simulink model "Navigation_loop_Animation"  (Simulink 8.5)
settings: Solver=ode45  StartTime=0.0  StopTime=20  RelTol=1e-3
values from neighbouring files (symbols this model uses):
  g = 9.8    [init_pararmeters.m]
  kdp = 0.4    [init_pararmeters.m]
  kdps = 0.4    [init_pararmeters.m]
  kdt = 0.4    [init_pararmeters.m]
  kdx = 0.5    [init_pararmeters.m]
  kdy = 0.5    [init_pararmeters.m]
  kdz = 20    [init_pararmeters.m]
  kix = 0    [init_pararmeters.m]
  kiy = 0    [init_pararmeters.m]
  kpp = 0.8    [init_pararmeters.m]
  kpps = 1    [init_pararmeters.m]
  kpt = 1.2    [init_pararmeters.m]
  kpx = 0.8    [init_pararmeters.m]
  kpy = 0.8    [init_pararmeters.m]
  kpz = 100    [init_pararmeters.m]
libraries: aerolibutil x2, vrlib x1
settings Model: Creator=abdelrazzak.merheb  LastModifiedBy=flying
settings DebuggingCC: SolverPrmCheckMsg=warning  FcnCallInpInsideContextMsg=UseLocalSettings

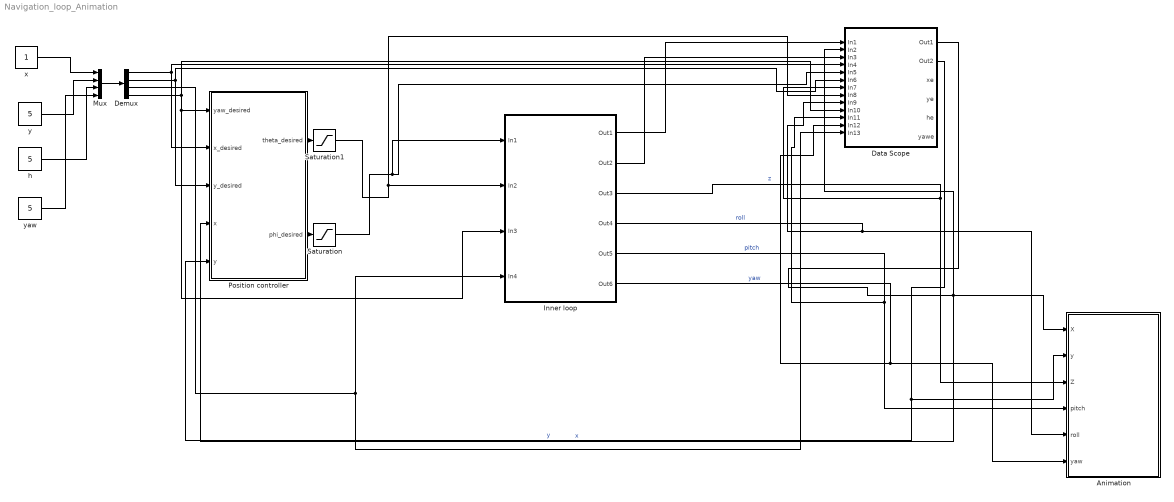
== system Navigation_loop_Animation ==
  "Animation " : Subsystem
  Data Scope : Subsystem
  Demux : Demux
  Inner loop : Subsystem
  Mux : Mux
  Position controller : Subsystem
  Saturation : Saturate  UpperLimit=35/57.3  LowerLimit=-35/57.3
  Saturation1 : Saturate  UpperLimit=35/57.3  LowerLimit=-35/57.3
  h : Constant  Value=5
  x : Constant
  y : Constant  Value=5
  yaw : Constant  Value=5
  wires:
  Demux/3 -> Inner loop/4(In4), Data Scope/13(In13)
  Demux/4 -> Data Scope/10(In10), Inner loop/3(In3), Position controller/1(yaw_desired)
  Demux/1 -> Data Scope/4(In4), Position controller/2(x_desired)
  Demux/2 -> Data Scope/6(In6), Position controller/3(y_desired)
  Saturation/1 -> Inner loop/1(In1), Data Scope/5(In5)
  Saturation1/1 -> Data Scope/8(In8), Inner loop/2(In2)
  Position controller/1(theta_desired) -> Saturation1/1
  Position controller/2(phi_desired) -> Saturation/1
  Data Scope/1(Out1) -> "Animation "/1(X), Data Scope/2(In2), Position controller/4(x)  "x"
  Data Scope/2(Out2) -> Position controller/5(y), "Animation "/2(y)  "y"
  Inner loop/5(Out5) -> "Animation "/4(pitch), Data Scope/11(In11)  "pitch"
  Inner loop/3(Out3) -> "Animation "/3(Z), Data Scope/7(In7)  "z"
  Inner loop/4(Out4) -> "Animation "/5(roll), Data Scope/9(In9)  "roll"
  Inner loop/6(Out6) -> "Animation "/6(yaw), Data Scope/12(In12)  "yaw"
  Inner loop/1(Out1) -> Data Scope/1(In1)
  Inner loop/2(Out2) -> Data Scope/3(In3)
  Mux/1 -> Demux/1
  x/1 -> Mux/1
  y/1 -> Mux/2
  h/1 -> Mux/3
  yaw/1 -> Mux/4

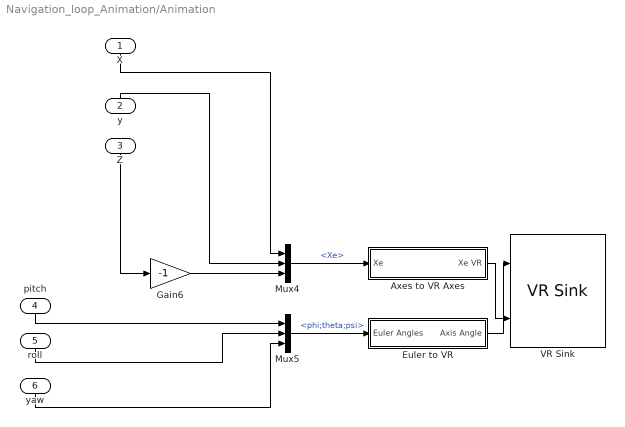
== system Navigation_loop_Animation/Animation  ==
  X : Inport
  y : Inport  Port=2
  Z : Inport  Port=3
  pitch : Inport  Port=4
  roll : Inport  Port=5
  yaw : Inport  Port=6
  Axes to VR Axes : Subsystem
  Euler to VR : Subsystem
  Gain6 : Gain  Gain=-1
  Mux4 : Mux  Inputs=3
  Mux5 : Mux  Inputs=3
  VR Sink : vrlib/VR Sink  InstantiateOnLoad=on  SampleTime=0.1  ViewEnable=on  RemoteChange=off  RemoteView=on  FieldsWritten=MyAirCraft.rotation.4.1.1.double#MyAirCraft.translation.3.1.1.double  WorldFileName=rollTst.wrl  AutoView=off  VideoDimensions=[]  AllowVariableSize=off
  wires:
  Mux5/1 -> Euler to VR/1(Euler Angles)  "<phi;theta;psi>"
  Gain6/1 -> Mux4/3
  Axes to VR Axes/1(Xe VR) -> VR Sink/2
  Euler to VR/1(Axis Angle) -> VR Sink/1
  Mux4/1 -> Axes to VR Axes/1(Xe)  "<Xe>"
  yaw/1 -> Mux5/3
  roll/1 -> Mux5/2
  y/1 -> Mux4/2
  pitch/1 -> Mux5/1
  Z/1 -> Gain6/1
  X/1 -> Mux4/1

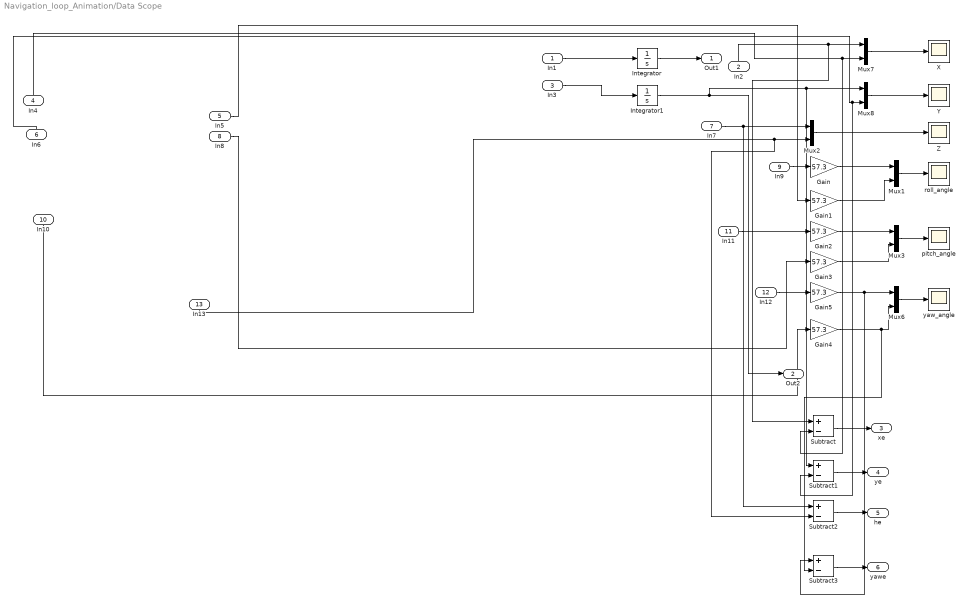
== system Navigation_loop_Animation/Data Scope ==
  In1 : Inport
  In2 : Inport  Port=2
  In3 : Inport  Port=3
  In4 : Inport  Port=4
  In5 : Inport  Port=5
  In6 : Inport  Port=6
  In7 : Inport  Port=7
  In8 : Inport  Port=8
  In9 : Inport  Port=9
  In10 : Inport  Port=10
  In11 : Inport  Port=11
  In12 : Inport  Port=12
  In13 : Inport  Port=13
  Gain{,1..5} (6 alike) : Gain  Gain=57.3
  Integrator : Integrator
  Integrator1 : Integrator
  Mux{1..3,6..8} (6 alike) : Mux  Inputs=2
  Subtract{,1..3} (4 alike) : Sum  Inputs=+-
  X : Scope
      settings: YMin=9.50171  YMax=10.5019
  Y : Scope
      settings: YMin=-53000  YMax=-50750  SaveName=ScopeData2
  Z : Scope
      settings: YMin=95  YMax=105  SaveName=ScopeData3
  pitch_angle : Scope
  roll_angle : Scope
      settings: YMax=20  SaveName=ScopeData4
  yaw_angle : Scope
      settings: YMin=-3.29867  YMax=-2.98451  SaveName=ScopeData5
  Out1 : Outport
  Out2 : Outport  Port=2
  xe : Outport  Port=3
  ye : Outport  Port=4
  he : Outport  Port=5
  yawe : Outport  Port=6
  wires:
  In1/1 -> Integrator/1
  Integrator1/1 -> Out2/1, Mux8/1, Subtract1/1
  Mux1/1 -> roll_angle/1
  In3/1 -> Integrator1/1
  Integrator/1 -> Out1/1
  Gain/1 -> Mux1/1
  Gain5/1 -> Subtract3/1, Mux6/1
  Gain4/1 -> Subtract3/2, Mux6/2
  Mux8/1 -> Y/1
  Mux7/1 -> X/1
  Gain3/1 -> Mux3/2
  Mux3/1 -> pitch_angle/1
  Mux2/1 -> Z/1
  Gain1/1 -> Mux1/2
  Gain2/1 -> Mux3/1
  Mux6/1 -> yaw_angle/1
  In12/1 -> Gain5/1
  In9/1 -> Gain/1
  In2/1 -> Subtract/1, Mux7/1
  In11/1 -> Gain2/1
  In8/1 -> Gain3/1
  In13/1 -> Subtract2/2, Mux2/2
  In5/1 -> Gain1/1
  In4/1 -> Subtract/2, Mux7/2
  In6/1 -> Subtract1/2, Mux8/2
  In7/1 -> Mux2/1, Subtract2/1
  In10/1 -> Gain4/1
  Subtract3/1 -> yawe/1
  Subtract2/1 -> he/1
  Subtract1/1 -> ye/1
  Subtract/1 -> xe/1

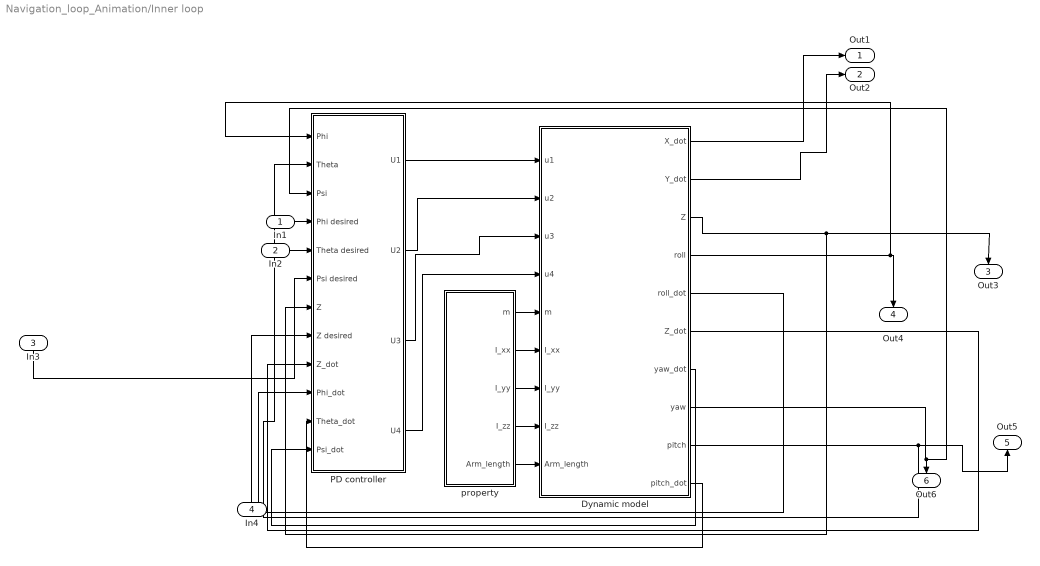
== system Navigation_loop_Animation/Inner loop ==
  In1 : Inport
  In2 : Inport  Port=2
  In3 : Inport  Port=3
  In4 : Inport  Port=4
  Dynamic model : Subsystem
  PD controller : Subsystem
  "property " : Subsystem
  Out1 : Outport
  Out2 : Outport  Port=2
  Out3 : Outport  Port=3
  Out4 : Outport  Port=4
  Out5 : Outport  Port=5
  Out6 : Outport  Port=6
  wires:
  Dynamic model/9(pitch) -> Out5/1, PD controller/2(Theta)
  Dynamic model/3(Z) -> Out3/1, PD controller/7(Z)
  PD controller/2(U2) -> Dynamic model/2(u2)
  PD controller/3(U3) -> Dynamic model/3(u3)
  PD controller/1(U1) -> Dynamic model/1(u1)
  PD controller/4(U4) -> Dynamic model/4(u4)
  "property "/1(m) -> Dynamic model/5(m)
  "property "/2(I_xx) -> Dynamic model/6(I_xx)
  "property "/5("Arm_length ") -> Dynamic model/9(Arm_length)
  Dynamic model/6(Z_dot) -> PD controller/9(Z_dot)
  Dynamic model/7(yaw_dot) -> PD controller/12("Psi_dot ")
  "property "/4(I_zz) -> Dynamic model/8(I_zz)
  Dynamic model/5(roll_dot) -> PD controller/10(Phi_dot)
  "property "/3(I_yy) -> Dynamic model/7(I_yy)
  Dynamic model/10(pitch_dot) -> PD controller/11(Theta_dot)
  Dynamic model/2(Y_dot) -> Out2/1
  Dynamic model/1("X_dot ") -> Out1/1
  In3/1 -> PD controller/6(Psi desired)
  In1/1 -> PD controller/4(Phi desired)
  Dynamic model/4(roll) -> Out4/1, PD controller/1(Phi)
  Dynamic model/8(yaw) -> PD controller/3(Psi), Out6/1
  In2/1 -> PD controller/5(Theta desired)
  In4/1 -> PD controller/8(Z desired)

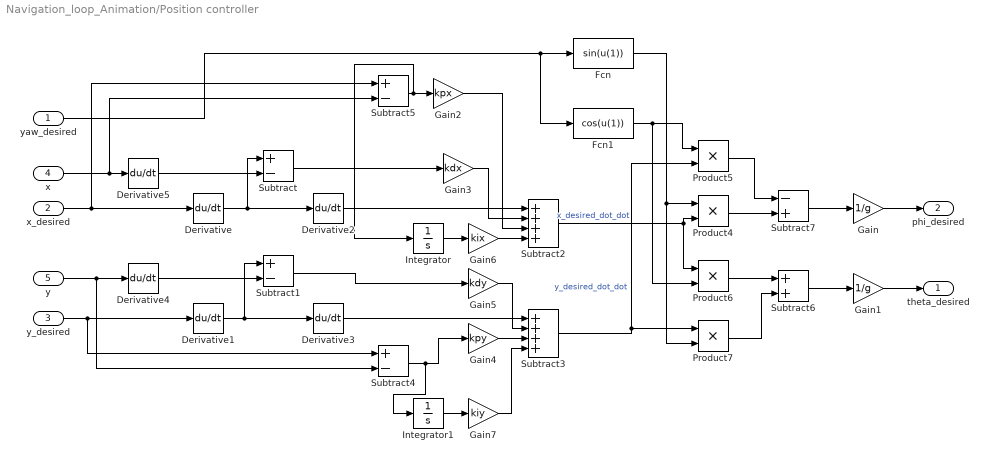
== system Navigation_loop_Animation/Position controller ==
  yaw_desired : Inport
  x_desired : Inport  Port=2
  y_desired : Inport  Port=3
  x : Inport  Port=4
  y : Inport  Port=5
  Derivative{,1..5} (6 alike) : Derivative
  Fcn : Fcn  Expr=sin(u(1))
  Fcn1 : Fcn  Expr=cos(u(1))
  Gain : Gain  Gain=1/g
  Gain1 : Gain  Gain=1/g
  Gain2 : Gain  Gain=kpx
  Gain3 : Gain  Gain=kdx
  Gain4 : Gain  Gain=kpy
  Gain5 : Gain  Gain=kdy
  Gain6 : Gain  Gain=kix
  Gain7 : Gain  Gain=kiy
  Integrator : Integrator
  Integrator1 : Integrator
  Product{4..7} (4 alike) : Product
  Subtract{,1,4..5} (4 alike) : Sum  Inputs=+-
  Subtract2 : Sum  Inputs=++++
  Subtract3 : Sum  Inputs=++++
  Subtract6 : Sum
  Subtract7 : Sum  Inputs=-+
  theta_desired : Outport
  phi_desired : Outport  Port=2
  wires:
  Subtract4/1 -> Gain4/1, Integrator1/1
  Integrator1/1 -> Gain7/1
  Integrator/1 -> Gain6/1
  Gain7/1 -> Subtract3/4
  Gain6/1 -> Subtract2/4
  Gain2/1 -> Subtract2/3
  Subtract5/1 -> Gain2/1, Integrator/1
  Fcn/1 -> Product4/1, Product7/2
  Gain1/1 -> theta_desired/1
  yaw_desired/1 -> Fcn/1, Fcn1/1
  Gain/1 -> phi_desired/1
  Product4/1 -> Subtract7/2
  Subtract1/1 -> Gain5/1
  Fcn1/1 -> Product5/1, Product6/2
  Subtract7/1 -> Gain/1
  Gain3/1 -> Subtract2/2
  Product5/1 -> Subtract7/1
  Derivative3/1 -> Subtract3/1
  Subtract6/1 -> Gain1/1
  Product7/1 -> Subtract6/2
  Product6/1 -> Subtract6/1
  Derivative2/1 -> Subtract2/1
  y_desired/1 -> Derivative1/1, Subtract4/1
  Derivative1/1 -> Derivative3/1, Subtract1/1
  x_desired/1 -> Derivative/1, Subtract5/1
  Derivative/1 -> Derivative2/1, Subtract/1
  Gain5/1 -> Subtract3/2
  Derivative5/1 -> Subtract/2
  x/1 -> Derivative5/1, Subtract5/2
  Derivative4/1 -> Subtract1/2
  y/1 -> Derivative4/1, Subtract4/2
  Subtract3/1 -> Product5/2, Product7/1  "y_desired_dot_dot"
  Gain4/1 -> Subtract3/3
  Subtract2/1 -> Product4/2, Product6/1  "x_desired_dot_dot"
  Subtract/1 -> Gain3/1

== system Navigation_loop_Animation/Animation /Axes to VR Axes ==
  Xe : Inport
  Demux : Demux  Outputs=3
  Mux : Mux  Inputs=3
  rad-->deg : Gain  Gain=-1  SaturateOnIntegerOverflow=on  OutDataTypeStr=Inherit: Same as input  ParamDataTypeStr=Inherit: Same as input
  rad-->deg1 : Gain  Gain=-1  SaturateOnIntegerOverflow=on  OutDataTypeStr=Inherit: Same as input  ParamDataTypeStr=Inherit: Same as input
  Xe VR : Outport
  wires:
  Xe/1 -> Demux/1
  Demux/1 -> Mux/1
  Demux/2 -> rad-->deg/1
  Demux/3 -> rad-->deg1/1
  Mux/1 -> Xe VR/1
  rad-->deg1/1 -> Mux/2
  rad-->deg/1 -> Mux/3

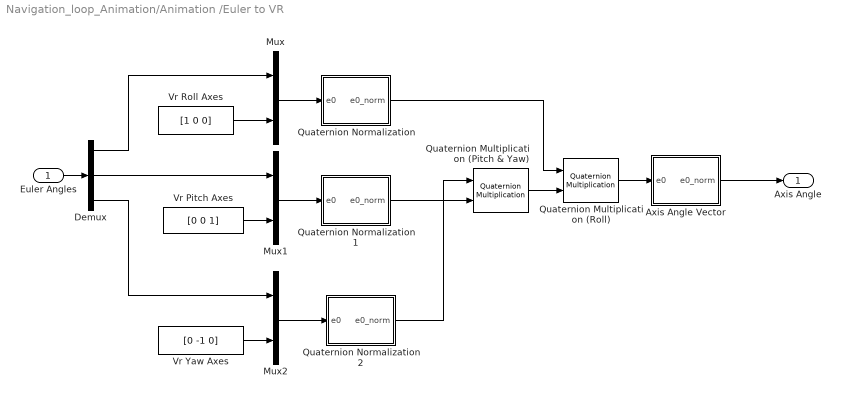
== system Navigation_loop_Animation/Animation /Euler to VR ==
  Euler Angles : Inport
  Axis Angle Vector : Subsystem
  Demux : Demux  Outputs=3
  Mux : Mux  Inputs=2
  Mux1 : Mux  Inputs=2
  Mux2 : Mux  Inputs=2
  Quaternion Multiplication (Pitch & Yaw) : aerolibutil/Quaternion Multiplication
  Quaternion Multiplication (Roll) : aerolibutil/Quaternion Multiplication
  Quaternion Normalization : Subsystem
  Quaternion Normalization1 : Subsystem
  Quaternion Normalization2 : Subsystem
  Vr Pitch Axes : Constant  Value=[0 0 1]
  Vr Roll Axes : Constant  Value=[1 0 0]
  Vr Yaw Axes : Constant  Value=[0 -1 0]
  Axis Angle : Outport
  wires:
  Quaternion Multiplication (Roll)/1 -> Axis Angle Vector/1(e0)
  Quaternion Multiplication (Pitch & Yaw)/1 -> Quaternion Multiplication (Roll)/2
  Axis Angle Vector/1(e0_norm) -> Axis Angle/1
  Quaternion Normalization/1(e0_norm) -> Quaternion Multiplication (Roll)/1
  Quaternion Normalization2/1(e0_norm) -> Quaternion Multiplication (Pitch & Yaw)/1
  Quaternion Normalization1/1(e0_norm) -> Quaternion Multiplication (Pitch & Yaw)/2
  Mux2/1 -> Quaternion Normalization2/1(e0)
  Mux1/1 -> Quaternion Normalization1/1(e0)
  Mux/1 -> Quaternion Normalization/1(e0)
  Demux/3 -> Mux2/1
  Vr Yaw Axes/1 -> Mux2/2
  Demux/2 -> Mux1/1
  Vr Pitch Axes/1 -> Mux1/2
  Demux/1 -> Mux/1
  Vr Roll Axes/1 -> Mux/2
  Euler Angles/1 -> Demux/1

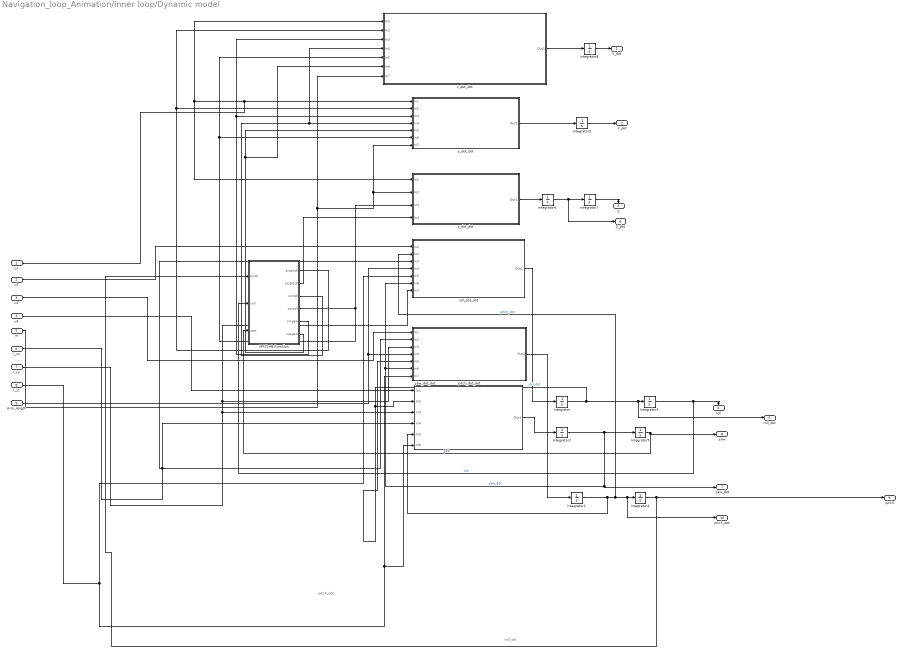
== system Navigation_loop_Animation/Inner loop/Dynamic model ==
  note: pitch_dot
  note: roll_dot
  u1 : Inport
  u2 : Inport  Port=2
  u3 : Inport  Port=3
  u4 : Inport  Port=4
  m : Inport  Port=5
  I_xx : Inport  Port=6
  I_yy : Inport  Port=7
  I_zz : Inport  Port=8
  Arm_length : Inport  Port=9
  Integrator{,1..9} (10 alike) : Integrator
  MATLAB Function : MATLAB Function  TreatAsAtomicUnit=on
  pitch_dot_dot : Subsystem
  roll_dot_dot : Subsystem
  x_dot_dot : Subsystem
  y_dot_dot : Subsystem
  yaw_dot_dot : Subsystem
  z_dot_dot : Subsystem
  "X_dot " : Outport
  Y_dot : Outport  Port=2
  Z : Outport  Port=3
  roll : Outport  Port=4
  roll_dot : Outport  Port=5
  Z_dot : Outport  Port=6
  yaw_dot : Outport  Port=7
  yaw : Outport  Port=8
  pitch : Outport  Port=9
  pitch_dot : Outport  Port=10
  wires:
  x_dot_dot/1(Out1) -> Integrator8/1
  Integrator6/1 -> Integrator7/1, Z_dot/1
  u4/1 -> yaw_dot_dot/1(In1)
  MATLAB Function/6(cosyaw) -> x_dot_dot/6(In6), y_dot_dot/5(In5)
  MATLAB Function/3(sinroll) -> x_dot_dot/4(In4), y_dot_dot/4(In4)
  MATLAB Function/4(cosroll) -> x_dot_dot/5(In5), y_dot_dot/6(In6), z_dot_dot/3(In3)
  MATLAB Function/1(sinpitch) -> x_dot_dot/2(In2), y_dot_dot/2(In2)
  m/1 -> x_dot_dot/7(In7), z_dot_dot/2(In2), y_dot_dot/7(In7)
  MATLAB Function/5(sinyaw) -> x_dot_dot/3(In3), y_dot_dot/3(In3)
  u1/1 -> y_dot_dot/1(In1), x_dot_dot/1(In1), z_dot_dot/1(In1)
  I_xx/1 -> yaw_dot_dot/4(In4), roll_dot_dot/3(In3), pitch_dot_dot/2(In2)
  I_yy/1 -> yaw_dot_dot/3(In3), roll_dot_dot/7(In7), pitch_dot_dot/3(In3)
  I_zz/1 -> roll_dot_dot/5(In5), yaw_dot_dot/6(In6), pitch_dot_dot/7(In7)
  Integrator3/1 -> roll/1, MATLAB Function/2(roll)  "roll"
  Integrator1/1 -> yaw_dot_dot/5(In5), roll_dot_dot/2(In2), pitch_dot/1, Integrator4/1  "pitch_dot"
  Integrator2/1 -> roll_dot_dot/6(In6), pitch_dot_dot/6(In6), yaw_dot/1, Integrator5/1  "yaw_dot"
  Integrator/1 -> pitch_dot_dot/5(In5), yaw_dot_dot/2(In2), roll_dot/1, Integrator3/1  "roll_dot"
  Integrator8/1 -> "X_dot "/1
  Integrator9/1 -> Y_dot/1
  Integrator5/1 -> MATLAB Function/3(yaw), yaw/1  "yaw"
  z_dot_dot/1(Out1) -> Integrator6/1
  roll_dot_dot/1(Out1) -> Integrator/1
  pitch_dot_dot/1(Out1) -> Integrator1/1
  MATLAB Function/2(cospitch) -> z_dot_dot/4(In4)
  u2/1 -> roll_dot_dot/1(In1)
  Arm_length/1 -> roll_dot_dot/4(In4), pitch_dot_dot/4(In4)
  u3/1 -> pitch_dot_dot/1(In1)
  y_dot_dot/1(Out1) -> Integrator9/1
  Integrator4/1 -> pitch/1, MATLAB Function/1(pitch)
  Integrator7/1 -> Z/1
  yaw_dot_dot/1(Out1) -> Integrator2/1

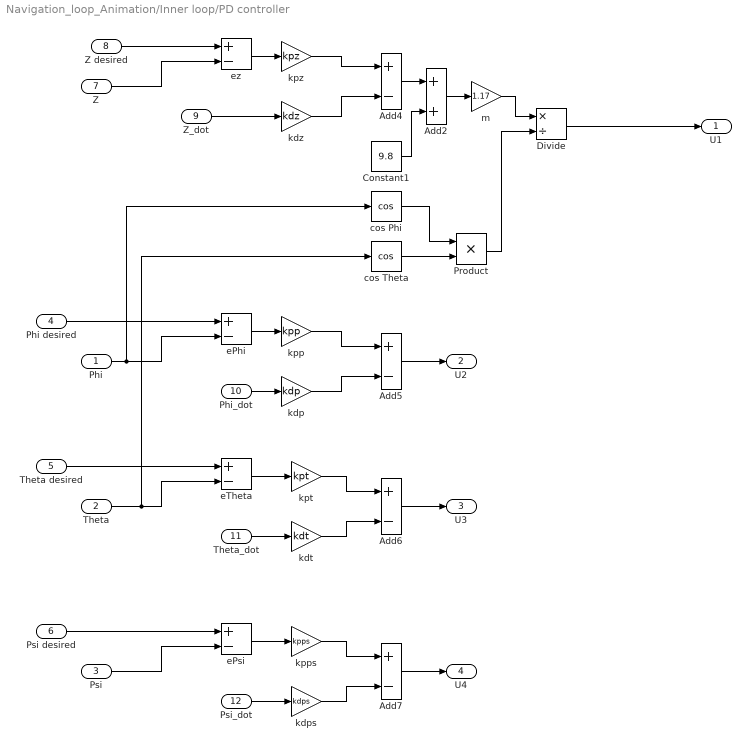
== system Navigation_loop_Animation/Inner loop/PD controller ==
  Phi : Inport
  Theta : Inport  Port=2
  Psi : Inport  Port=3
  Phi desired : Inport  Port=4
  Theta desired : Inport  Port=5
  Psi desired : Inport  Port=6
  Z : Inport  Port=7
  Z desired : Inport  Port=8
  Z_dot : Inport  Port=9
  Phi_dot : Inport  Port=10
  Theta_dot : Inport  Port=11
  "Psi_dot " : Inport  Port=12
  Add2 : Sum
  Add{4..7} (4 alike) : Sum  Inputs=+-
  Constant1 : Constant  Value=9.8
  Divide : Product  Inputs=*/
  Product : Product  RndMeth=Zero
  cos Phi : Trigonometry  Operator=cos
  cos Theta : Trigonometry  Operator=cos
  ePhi : Sum  Inputs=+-
  ePsi : Sum  Inputs=+-
  eTheta : Sum  Inputs=+-
  ez : Sum  Inputs=+-
  kdp : Gain  Gain=kdp
  kdps : Gain  Gain=kdps
  kdt : Gain  Gain=kdt
  kdz : Gain  Gain=kdz
  kpp : Gain  Gain=kpp
  kpps : Gain  Gain=kpps
  kpt : Gain  Gain=kpt
  kpz : Gain  Gain=kpz
  m : Gain  Gain=1.17
  U1 : Outport
  U2 : Outport  Port=2
  U3 : Outport  Port=3
  U4 : Outport  Port=4
  wires:
  Phi/1 -> ePhi/2, cos Phi/1
  Theta/1 -> eTheta/2, cos Theta/1
  Psi/1 -> ePsi/2
  Phi desired/1 -> ePhi/1
  Theta desired/1 -> eTheta/1
  Psi desired/1 -> ePsi/1
  ePhi/1 -> kpp/1
  Phi_dot/1 -> kdp/1
  eTheta/1 -> kpt/1
  Theta_dot/1 -> kdt/1
  ePsi/1 -> kpps/1
  "Psi_dot "/1 -> kdps/1
  Z desired/1 -> ez/1
  ez/1 -> kpz/1
  Z_dot/1 -> kdz/1
  kpz/1 -> Add4/1
  kdz/1 -> Add4/2
  kpp/1 -> Add5/1
  kdp/1 -> Add5/2
  Add5/1 -> U2/1
  kpt/1 -> Add6/1
  kdt/1 -> Add6/2
  Add6/1 -> U3/1
  kpps/1 -> Add7/1
  kdps/1 -> Add7/2
  Add7/1 -> U4/1
  cos Phi/1 -> Product/1
  cos Theta/1 -> Product/2
  m/1 -> Divide/1
  Product/1 -> Divide/2
  Divide/1 -> U1/1
  Add4/1 -> Add2/1
  Add2/1 -> m/1
  Constant1/1 -> Add2/2
  Z/1 -> ez/2

== system Navigation_loop_Animation/Inner loop/property  ==
  Arm_length_ : Constant  Value=0.228
  ineretia_yy : Constant  Value=2.5955e-4
  inertia_xx : Constant  Value=2.754e-4
  inertia_zz : Constant  Value=5.7824e-5
  mass : Constant  Value=1.17
  m : Outport
  I_xx : Outport  Port=2
  I_yy : Outport  Port=3
  I_zz : Outport  Port=4
  "Arm_length " : Outport  Port=5
  wires:
  inertia_zz/1 -> I_zz/1
  Arm_length_/1 -> "Arm_length "/1
  ineretia_yy/1 -> I_yy/1
  mass/1 -> m/1
  inertia_xx/1 -> I_xx/1

== system Navigation_loop_Animation/Animation /Euler to VR/Axis Angle Vector ==
  e0 : Inport
  2 : Gain  Gain=2  SaturateOnIntegerOverflow=on  OutDataTypeStr=Inherit: Same as input  ParamDataTypeStr=Inherit: Same as input
  Concatenate : Concatenate
  Demux : Demux  Outputs=[1 3 ]
  Product : Product  Inputs=*/  SaturateOnIntegerOverflow=on  InputSameDT=on  OutDataTypeStr=Inherit: Same as first input
  Trigonometric Function : Trigonometry
  Trigonometric Function2 : Trigonometry  Operator=acos
  e0_norm : Outport
  wires:
  Demux/1 -> Trigonometric Function2/1
  Demux/2 -> Product/1
  Concatenate/1 -> e0_norm/1
  Product/1 -> Concatenate/1
  2/1 -> Concatenate/2
  Trigonometric Function/1 -> Product/2
  Trigonometric Function2/1 -> Trigonometric Function/1, 2/1
  e0/1 -> Demux/1

== system Navigation_loop_Animation/Animation /Euler to VR/Quaternion Normalization ==
  e0 : Inport
  1/2 : Gain  Gain=1/2  SaturateOnIntegerOverflow=on  OutDataTypeStr=Inherit: Same as input  ParamDataTypeStr=Inherit: Same as input
  Concatenate : Concatenate
  Demux : Demux  Outputs=[1 3]
  Product : Product  SaturateOnIntegerOverflow=on  InputSameDT=on  OutDataTypeStr=Inherit: Same as first input
  Trigonometric Function : Trigonometry
  Trigonometric Function1 : Trigonometry  Operator=cos
  e0_norm : Outport
  wires:
  Trigonometric Function1/1 -> Concatenate/1
  Demux/2 -> Product/2
  Demux/1 -> 1/2/1
  Concatenate/1 -> e0_norm/1
  Product/1 -> Concatenate/2
  Trigonometric Function/1 -> Product/1
  1/2/1 -> Trigonometric Function1/1, Trigonometric Function/1
  e0/1 -> Demux/1

== system Navigation_loop_Animation/Animation /Euler to VR/Quaternion Normalization1 ==
  e0 : Inport
  1/2 : Gain  Gain=1/2  SaturateOnIntegerOverflow=on  OutDataTypeStr=Inherit: Same as input  ParamDataTypeStr=Inherit: Same as input
  Concatenate : Concatenate
  Demux : Demux  Outputs=[1 3]
  Product : Product  SaturateOnIntegerOverflow=on  InputSameDT=on  OutDataTypeStr=Inherit: Same as first input
  Trigonometric Function : Trigonometry
  Trigonometric Function1 : Trigonometry  Operator=cos
  e0_norm : Outport
  wires:
  e0/1 -> Demux/1
  1/2/1 -> Trigonometric Function/1, Trigonometric Function1/1
  Trigonometric Function/1 -> Product/1
  Product/1 -> Concatenate/2
  Concatenate/1 -> e0_norm/1
  Demux/1 -> 1/2/1
  Demux/2 -> Product/2
  Trigonometric Function1/1 -> Concatenate/1

== system Navigation_loop_Animation/Animation /Euler to VR/Quaternion Normalization2 ==
  e0 : Inport
  1/2 : Gain  Gain=1/2  SaturateOnIntegerOverflow=on  OutDataTypeStr=Inherit: Same as input  ParamDataTypeStr=Inherit: Same as input
  Concatenate : Concatenate
  Demux : Demux  Outputs=[1 3]
  Product : Product  SaturateOnIntegerOverflow=on  InputSameDT=on  OutDataTypeStr=Inherit: Same as first input
  Trigonometric Function : Trigonometry
  Trigonometric Function1 : Trigonometry  Operator=cos
  e0_norm : Outport
  wires:
  Trigonometric Function1/1 -> Concatenate/1
  Demux/2 -> Product/2
  Demux/1 -> 1/2/1
  Concatenate/1 -> e0_norm/1
  Product/1 -> Concatenate/2
  Trigonometric Function/1 -> Product/1
  1/2/1 -> Trigonometric Function1/1, Trigonometric Function/1
  e0/1 -> Demux/1

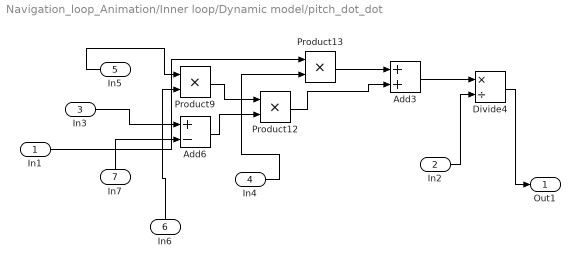
== system Navigation_loop_Animation/Inner loop/Dynamic model/pitch_dot_dot ==
  In1 : Inport
  In2 : Inport  Port=2
  In3 : Inport  Port=3
  In4 : Inport  Port=4
  In5 : Inport  Port=5
  In6 : Inport  Port=6
  In7 : Inport  Port=7
  Add3 : Sum
  Add6 : Sum  Inputs=+-
  Divide4 : Product  Inputs=*/
  Product12 : Product
  Product13 : Product
  Product9 : Product
  Out1 : Outport
  wires:
  Product12/1 -> Add3/2
  Product13/1 -> Add3/1
  In1/1 -> Product13/1
  Add6/1 -> Product12/2
  Add3/1 -> Divide4/1
  Product9/1 -> Product12/1
  In4/1 -> Product13/2
  In6/1 -> Product9/2
  In7/1 -> Add6/2
  In3/1 -> Add6/1
  In2/1 -> Divide4/2
  In5/1 -> Product9/1
  Divide4/1 -> Out1/1

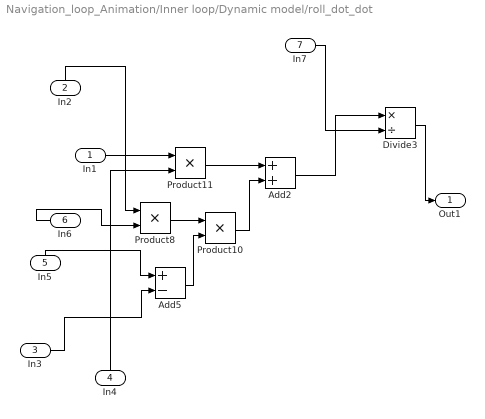
== system Navigation_loop_Animation/Inner loop/Dynamic model/roll_dot_dot ==
  In1 : Inport
  In2 : Inport  Port=2
  In3 : Inport  Port=3
  In4 : Inport  Port=4
  In5 : Inport  Port=5
  In6 : Inport  Port=6
  In7 : Inport  Port=7
  Add2 : Sum
  Add5 : Sum  Inputs=+-
  Divide3 : Product  Inputs=*/
  Product10 : Product
  Product11 : Product
  Product8 : Product
  Out1 : Outport
  wires:
  Product11/1 -> Add2/1
  Add5/1 -> Product10/2
  In1/1 -> Product11/1
  Add2/1 -> Divide3/1
  Product8/1 -> Product10/1
  Product10/1 -> Add2/2
  Divide3/1 -> Out1/1
  In5/1 -> Add5/1
  In3/1 -> Add5/2
  In2/1 -> Product8/1
  In7/1 -> Divide3/2
  In4/1 -> Product11/2
  In6/1 -> Product8/2

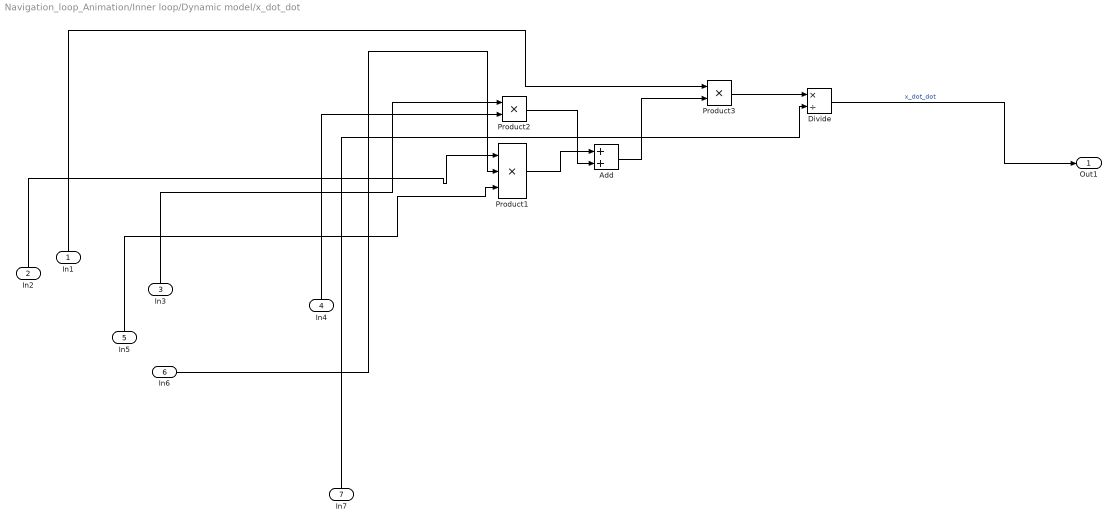
== system Navigation_loop_Animation/Inner loop/Dynamic model/x_dot_dot ==
  In1 : Inport
  In2 : Inport  Port=2
  In3 : Inport  Port=3
  In4 : Inport  Port=4
  In5 : Inport  Port=5
  In6 : Inport  Port=6
  In7 : Inport  Port=7
  Add : Sum
  Divide : Product  Inputs=*/
  Product1 : Product  Inputs=3
  Product2 : Product
  Product3 : Product
  Out1 : Outport
  wires:
  In1/1 -> Product3/1
  In6/1 -> Product1/2
  In7/1 -> Divide/2
  In4/1 -> Product2/2
  In3/1 -> Product2/1
  In5/1 -> Product1/3
  In2/1 -> Product1/1
  Divide/1 -> Out1/1  "x_dot_dot"
  Product2/1 -> Add/2
  Product1/1 -> Add/1
  Product3/1 -> Divide/1
  Add/1 -> Product3/2

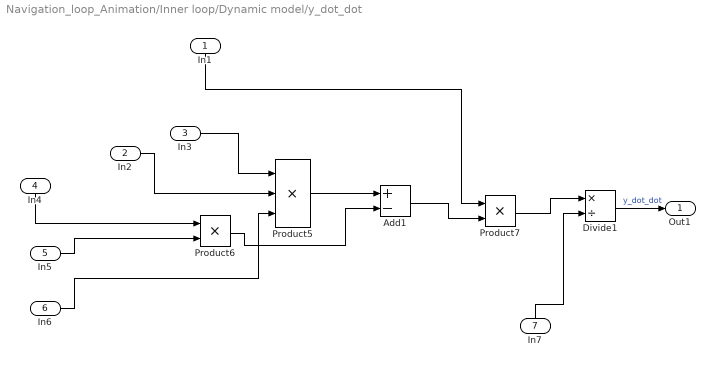
== system Navigation_loop_Animation/Inner loop/Dynamic model/y_dot_dot ==
  In1 : Inport
  In2 : Inport  Port=2
  In3 : Inport  Port=3
  In4 : Inport  Port=4
  In5 : Inport  Port=5
  In6 : Inport  Port=6
  In7 : Inport  Port=7
  Add1 : Sum  Inputs=+-
  Divide1 : Product  Inputs=*/
  Product5 : Product  Inputs=3
  Product6 : Product
  Product7 : Product
  Out1 : Outport
  wires:
  In1/1 -> Product7/1
  In2/1 -> Product5/2
  In5/1 -> Product6/2
  In7/1 -> Divide1/2
  In6/1 -> Product5/3
  In3/1 -> Product5/1
  In4/1 -> Product6/1
  Product5/1 -> Add1/1
  Add1/1 -> Product7/2
  Product6/1 -> Add1/2
  Divide1/1 -> Out1/1  "y_dot_dot"
  Product7/1 -> Divide1/1

== system Navigation_loop_Animation/Inner loop/Dynamic model/yaw_dot_dot ==
  In1 : Inport
  In2 : Inport  Port=2
  In3 : Inport  Port=3
  In4 : Inport  Port=4
  In5 : Inport  Port=5
  In6 : Inport  Port=6
  Add7 : Sum
  Add8 : Sum  Inputs=+-
  Divide5 : Product  Inputs=*/
  Product14 : Product
  Product15 : Product
  Out1 : Outport
  wires:
  In4/1 -> Add8/1
  In6/1 -> Divide5/2
  In2/1 -> Product15/2
  In3/1 -> Add8/2
  In5/1 -> Product15/1
  Product14/1 -> Add7/2
  Add8/1 -> Product14/2
  Product15/1 -> Product14/1
  In1/1 -> Add7/1
  Add7/1 -> Divide5/1
  Divide5/1 -> Out1/1

== system Navigation_loop_Animation/Inner loop/Dynamic model/z_dot_dot ==
  In1 : Inport
  In2 : Inport  Port=2
  In3 : Inport  Port=3
  In4 : Inport  Port=4
  Add4 : Sum  Inputs=-+
  Divide2 : Product  Inputs=*/
  Product : Product
  Product4 : Product
  u5 : Constant  Value=9.8
  Out1 : Outport
  wires:
  In3/1 -> Product4/2
  In2/1 -> Divide2/2
  In1/1 -> Product/2
  Divide2/1 -> Add4/2
  Product4/1 -> Product/1
  In4/1 -> Product4/1
  u5/1 -> Add4/1
  Product/1 -> Divide2/1
  Add4/1 -> Out1/1  "z_dot_dot"

== matlab function Inner loop/Dynamic model/MATLAB Function ==
  data: pitch input double; sinpitch output double; roll input double; yaw input double; cospitch output double; sinroll output double; cosroll output double; sinyaw output double; cosyaw output double
function [sinpitch,cospitch,sinroll,cosroll,sinyaw,cosyaw]= fcn(pitch,roll,yaw)
sinpitch=sin(pitch);
cospitch=cos(pitch);
sinroll=sin(roll);
cosroll=cos(roll);
sinyaw=sin(yaw);
cosyaw=cos(yaw);
